simulink model "ADC_withDither"  (R2012b)
settings: Solver=ode45  StartTime=0.0  StopTime=inf  RelTol=1e-3
libraries: simulink x1
settings Model: Creator=ayush  LastModifiedBy=ayush

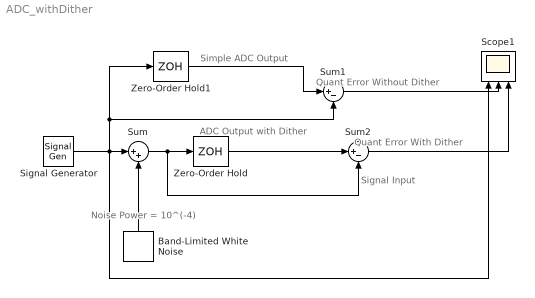
== system ADC_withDither ==
  note: Noise Power = 10^(-4)
  note: ADC Output with Dither
  note: Quant Error With Dither
  note: Signal Input
  note: Quant Error Without Dither
  note: Simple ADC Output
  Band-Limited White Noise : simulink/Sources/Band-Limited White Noise  Cov=[0.0001]  Ts=1/100  seed=[1]
  Scope1 : Scope  NumInputPorts=3
      settings: ShowLegends=on  TimeRange=0.1  YMin=-1~-1~-1.5  YMax=1~1~1.5  SampleInput=on
  Signal Generator : SignalGenerator  Frequency=100
  Sum : Sum  Inputs=|++
  Sum1 : Sum  Inputs=|+-
  Sum2 : Sum  Inputs=|+-
  Zero-Order Hold : ZeroOrderHold  SampleTime=1/5000
  Zero-Order Hold1 : ZeroOrderHold  SampleTime=1/5000
  wires:
  Zero-Order Hold/1 -> Sum2/1
  Signal Generator/1 -> Scope1/1, Sum1/2, Zero-Order Hold1/1, Sum/1
  Sum/1 -> Zero-Order Hold/1, Sum2/2
  Band-Limited White Noise/1 -> Sum/2
  Zero-Order Hold1/1 -> Sum1/1
  Sum1/1 -> Scope1/2
  Sum2/1 -> Scope1/3
